simulink model "pre_gumaka"  (R2022a)
settings: Solver=VariableStepAuto  StartTime=0.0  StopTime=10.0  RelTol=1e-3
values from neighbouring files (symbols this model uses):
  ki = Pop(i,3)    [fitness.m]    (also in gen3.m = best_ch(3,end); params.m = 0.1629)
  Vi = Pop(i,2)    [fitness.m]    (also in gen3.m = best_ch(2,end); params.m = 139.094)
undefined symbols (not defined in the file or in its folder): T1
settings Model: Creator=DFUNDO  LastModifiedBy=DFUNDO
settings ModelReferenceCC: EnableRefExpFcnMdlSchedulingChecks=off
settings RTWCC: Description=Generic Real-Time Target

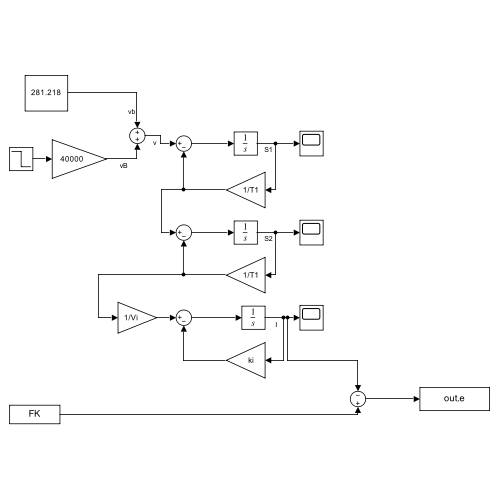
[thumbnail: Simulink's stored preview of the top-level diagram]
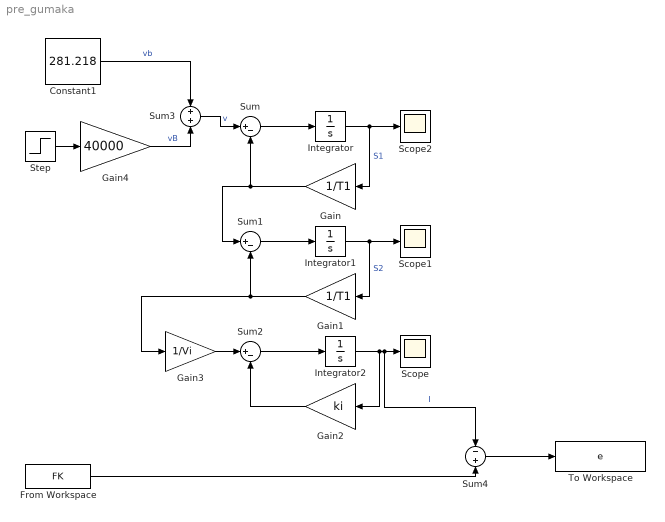
== system pre_gumaka ==
  Constant1 : Constant  Value=281.218
  From Workspace : FromWorkspace  VariableName=FK
  Gain : Gain  Gain=1/T1
  Gain1 : Gain  Gain=1/T1
  Gain2 : Gain  Gain=ki
  Gain3 : Gain  Gain=1/Vi
  Gain4 : Gain  Gain=40000
  Integrator : Integrator
  Integrator1 : Integrator
  Integrator2 : Integrator
  Scope : Scope
  Scope1 : Scope
  Scope2 : Scope
  Step : Step  Time=300  Before=1  After=0  SampleTime=0
  Sum : Sum  Inputs=|+-
  Sum1 : Sum  Inputs=|+-
  Sum2 : Sum  Inputs=|+-
  Sum3 : Sum
  Sum4 : Sum  Inputs=-+
  To Workspace : ToWorkspace  VariableName=e  SaveFormat=Timeseries  SampleTime=-1
  wires:
  Integrator/1 -> Gain/1, Scope2/1  "S1"
  Gain/1 -> Sum/2, Sum1/1
  Sum/1 -> Integrator/1
  Sum3/1 -> Sum/1  "v"
  Integrator1/1 -> Scope1/1, Gain1/1  "S2"
  Gain1/1 -> Gain3/1, Sum1/2
  Sum1/1 -> Integrator1/1
  Sum2/1 -> Integrator2/1
  Gain2/1 -> Sum2/2
  Integrator2/1 -> Gain2/1, Sum4/1, Scope/1  "I"
  Gain3/1 -> Sum2/1
  Constant1/1 -> Sum3/1  "vb"
  Gain4/1 -> Sum3/2  "vB"
  Step/1 -> Gain4/1
  From Workspace/1 -> Sum4/2
  Sum4/1 -> To Workspace/1
